simulink model "TFMMIoTSimAR"  (R2019b)
settings: Solver=VariableStepAuto  StartTime=0.0  StopTime=10  RelTol=1e-3
StartFcn:
  | startTimeStamp = num2str(posixtime(datetime('now')) * 1e6);
  | disp(strcat("Script Start: ", startTimeStamp));
  | cont = 0;
StopFcn:
  | topicMovAux = strcat(topicMov, "/Details");
  | timeStamp = num2str(posixtime(datetime('now')) * 1e6);
  | disp(strcat("Script End: ", timeStamp));
  | 
  | %Mensaje: CodigoEntrenamiento CodigoMovimiento FechaInicio FechaFin
  | msg = strcat(num2str(movCodeTrain), " ", num2str(movCode), " ", startTimeStamp, " ", timeStamp);
  | 
  | if movCodeTrain == 3
  |     msg = strcat(msg, " ", num2str(messValue));
  | end
  | 
  | publish(myMQTT, topicMovAux, msg);
model workspace (MAT data in the model file):
  gen3 = robotics.RigidBodyTree
  gen3.TreeInternal = robotics.manip.internal.RigidBodyTree
  gen3.TreeInternal.NumBodies = 8
  gen3.TreeInternal.Base = robotics.manip.internal.RigidBody
  gen3.TreeInternal.Base.Index = 0
  gen3.TreeInternal.Base.NameInternal = 'base_link'
  gen3.TreeInternal.Base.JointInternal = robotics.Joint
  gen3.TreeInternal.Base.JointInternal.Type = 'fixed'
  gen3.TreeInternal.Base.JointInternal.VelocityNumber = 0
  gen3.TreeInternal.Base.JointInternal.PositionNumber = 0
  gen3.TreeInternal.Base.JointInternal.MotionSubspace = [0; 0; 0; 0; 0; 0]
  gen3.TreeInternal.Base.JointInternal.NameInternal = 'base_link_jnt'
  gen3.TreeInternal.Base.ParentIndex = -1
  gen3.TreeInternal.Base.ChildrenIndices = 1
  gen3.TreeInternal.Base.MassInternal = 1.661
  gen3.TreeInternal.Base.CenterOfMassInternal = [-0.00077898 -4.2629e-05 0.077301]
  gen3.TreeInternal.Base.InertiaInternal = [0.0146026165007  -3.37077056916e-07  5.17806646798e-05; -3.37077056916e-07  0.0146456213934  1.24353405047e-06; 5.17806646798e-05  1.24353405047e-06  0.00199681092957]
  gen3.TreeInternal.Base.SpatialInertia = [0.0146026165007  -3.37077056916e-07  5.17806646798e-05  0  -0.128396961  -7.0806769e-05; -3.37077056916e-07  0.0146456213934  1.24353405047e-06  0.128396961  0  0.00129388578; 5.17806646798e-05  1.24353405047e-06  0.00199681092957  7.0806769e-05  -0.00129388578  0; 0  0.128396961  7.0806769e-05  1.661  0  0; -0.128396961  0  -0.00129388578  0  1.661  0; -7.0806769e-05  0.00129388578  0  0  0  1.661]
  gen3.TreeInternal.Base.VisualsInternal{1} = robotics.manip.internal.RigidBodyGeometry
  gen3.TreeInternal.Base.VisualsInternal{1}.SourceData = {'Mesh', '/mathworks/devel/bat/Brobot/build/matlab/toolbox/robotics/robotmanip/data/kortex_description/meshes/base_link.STL'}
  gen3.TreeInternal.Base.VisualsInternal{1}.Vertices = [0.0238897390664 0.0238897390664 0.0248048026115 0.0248048026115 0.0260548014194 0.0260548014194 0.0273048020899 0.0273048020899 0.028219865635 0.028219865635 0.0285465624183 0.0285548008978 ... (5268 elements, 1756x3)]
  gen3.TreeInternal.Base.VisualsInternal{1}.Faces = [1 3 3 5 5 7 7 8 9 9 12 12 ... (10362 elements, 3454x3)]
  gen3.TreeInternal.Base.VisualsInternal{1}.Color = [0.79216 0.81961 0.93333 1]
  gen3.TreeInternal.Base.VisualsInternal{1}.Tform = [1  0  0  0; 0  1  0  0; 0  0  1  0; 0  0  0  1]
  gen3.TreeInternal.Gravity = [0 0 -9.81]
  gen3.TreeInternal.Bodies{1} = robotics.manip.internal.RigidBody
  gen3.TreeInternal.Bodies{1}.Index = 1
  gen3.TreeInternal.Bodies{1}.NameInternal = 'Shoulder_Link'
  gen3.TreeInternal.Bodies{1}.JointInternal = robotics.Joint
  gen3.TreeInternal.Bodies{1}.JointInternal.Type = 'revolute'
  gen3.TreeInternal.Bodies{1}.JointInternal.VelocityNumber = 1
  gen3.TreeInternal.Bodies{1}.JointInternal.PositionNumber = 1
  gen3.TreeInternal.Bodies{1}.JointInternal.MotionSubspace = [0; 0; 1; 0; 0; 0]
  gen3.TreeInternal.Bodies{1}.JointInternal.InTree = 1
  gen3.TreeInternal.Bodies{1}.JointInternal.JointToParentTransform = [1  0  0  0; 0  -0.999999999973  7.34641020664e-06  0; 0  -7.34641020664e-06  -0.999999999973  0.15643; 0  0  0  1]
  gen3.TreeInternal.Bodies{1}.JointInternal.NameInternal = 'Actuator1'
  gen3.TreeInternal.Bodies{1}.JointInternal.PositionLimitsInternal = [-Inf Inf]
  gen3.TreeInternal.Bodies{1}.JointInternal.JointAxisInternal = [0 0 1]
  gen3.TreeInternal.Bodies{1}.ParentIndex = 0
  gen3.TreeInternal.Bodies{1}.ChildrenIndices = [0 1]
  gen3.TreeInternal.Bodies{1}.MassInternal = 2.009
  gen3.TreeInternal.Bodies{1}.CenterOfMassInternal = [-2.2888e-05 -0.010511 -0.075159]
  gen3.TreeInternal.Bodies{1}.InertiaInternal = [0.0160786470116  -1.34157671791e-06  -5.35566053673e-06; -1.34157671791e-06  0.016118091492  -0.00204244246424; -5.35566053673e-06  -0.00204244246424  0.00161225762452]
  gen3.TreeInternal.Bodies{1}.SpatialInertia = [0.0160786470116  -1.34157671791e-06  -5.35566053673e-06  0  0.150994431  -0.021116599; -1.34157671791e-06  0.016118091492  -0.00204244246424  -0.150994431  0  4.5981992e-05; -5.35566053673e-06  -0.00204244246424  0.00161225762452  0.021116599  -4.5981992e-05  0; 0  -0.150994431  0.021116599  2.009  0  0; 0.150994431  0  -4.5981992e-05  0  2.009  0; -0.021116599  4.5981992e-05  0  0  0  2.009]
  gen3.TreeInternal.Bodies{1}.VisualsInternal{1} = robotics.manip.internal.RigidBodyGeometry
  gen3.TreeInternal.Bodies{1}.VisualsInternal{1}.SourceData = {'Mesh', '/mathworks/devel/bat/Brobot/build/matlab/toolbox/robotics/robotmanip/data/kortex_description/meshes/Shoulder_Link.STL'}
  gen3.TreeInternal.Bodies{1}.VisualsInternal{1}.Vertices = [-0.00565051892772 0.000944308878388 0.000944308878388 0.00751337828115 0.00751337828115 0.0138775017112 0.0138775017112 0.0198630858213 0.0198630858213 0.0253068543971 0.0253068543971 0.03006031923 ... (14295 elements, 4765x3)]
  gen3.TreeInternal.Bodies{1}.VisualsInternal{1}.Faces = [1 3 3 5 5 7 7 9 9 11 11 13 ... (28566 elements, 9522x3)]
  gen3.TreeInternal.Bodies{1}.VisualsInternal{1}.Color = [0.86667 0.86667 0.8902 1]
  gen3.TreeInternal.Bodies{1}.VisualsInternal{1}.Tform = [1  0  0  0; 0  1  0  0; 0  0  1  0; 0  0  0  1]
  gen3.TreeInternal.Bodies{2} = robotics.manip.internal.RigidBody
  gen3.TreeInternal.Bodies{2}.Index = 2
  gen3.TreeInternal.Bodies{2}.NameInternal = 'HalfArm1_Link'
  gen3.TreeInternal.Bodies{2}.JointInternal = robotics.Joint
  gen3.TreeInternal.Bodies{2}.JointInternal.Type = 'revolute'
  gen3.TreeInternal.Bodies{2}.JointInternal.VelocityNumber = 1
  gen3.TreeInternal.Bodies{2}.JointInternal.PositionNumber = 1
  gen3.TreeInternal.Bodies{2}.JointInternal.MotionSubspace = [0; 0; 1; 0; 0; 0]
  gen3.TreeInternal.Bodies{2}.JointInternal.InTree = 1
  gen3.TreeInternal.Bodies{2}.JointInternal.JointToParentTransform = [1  0  0  0; 0  -3.67320510335e-06  -0.999999999993  0.005375; 0  0.999999999993  -3.67320510335e-06  -0.12838; 0  0  0  1]
  gen3.TreeInternal.Bodies{2}.JointInternal.NameInternal = 'Actuator2'
  gen3.TreeInternal.Bodies{2}.JointInternal.PositionLimitsInternal = [-2.2 2.2]
  gen3.TreeInternal.Bodies{2}.JointInternal.JointAxisInternal = [0 0 1]
  gen3.TreeInternal.Bodies{2}.ParentIndex = 1
  gen3.TreeInternal.Bodies{2}.ChildrenIndices = [0 0 1]
  gen3.TreeInternal.Bodies{2}.MassInternal = 1.106
  gen3.TreeInternal.Bodies{2}.CenterOfMassInternal = [-2.7821e-05 -0.097298 -0.012693]
  gen3.TreeInternal.Bodies{2}.InertiaInternal = [0.0195653824366  -5.89336198975e-06  -5.56983940018e-07; -5.89336198975e-06  0.000909251003447  -0.000848233886484; -5.56983940018e-07  -0.000848233886484  0.0195119931453]
  gen3.TreeInternal.Bodies{2}.SpatialInertia = [0.0195653824366  -5.89336198975e-06  -5.56983940018e-07  0  0.014038458  -0.107611588; -5.89336198975e-06  0.000909251003447  -0.000848233886484  -0.014038458  0  3.0770026e-05; -5.56983940018e-07  -0.000848233886484  0.0195119931453  0.107611588  -3.0770026e-05  0; 0  -0.014038458  0.107611588  1.106  0  0; 0.014038458  0  -3.0770026e-05  0  1.106  0; -0.107611588  3.0770026e-05  0  0  0  1.106]
  gen3.TreeInternal.Bodies{2}.VisualsInternal{1} = robotics.manip.internal.RigidBodyGeometry
  gen3.TreeInternal.Bodies{2}.VisualsInternal{1}.SourceData = {'Mesh', '/mathworks/devel/bat/Brobot/build/matlab/toolbox/robotics/robotmanip/data/kortex_description/meshes/HalfArm1_Link.STL'}
  gen3.TreeInternal.Bodies{2}.VisualsInternal{1}.Vertices = [-0.00426170928404 -0.0107498951256 -0.0107498951256 -0.0169448517263 -0.0169448517263 -0.0226775947958 -0.0226775947958 -0.0277917552739 -0.0277917552739 -0.0321478284895 -0.0321478284895 -0.0356269925833 ... (15435 elements, 5145x3)]
  gen3.TreeInternal.Bodies{2}.VisualsInternal{1}.Faces = [1 3 3 5 5 7 7 9 9 11 11 13 ... (30846 elements, 10282x3)]
  gen3.TreeInternal.Bodies{2}.VisualsInternal{1}.Color = [0.89804 0.91765 0.92941 1]
  gen3.TreeInternal.Bodies{2}.VisualsInternal{1}.Tform = [1  0  0  0; 0  1  0  0; 0  0  1  0; 0  0  0  1]
  gen3.TreeInternal.Bodies{3} = robotics.manip.internal.RigidBody
  gen3.TreeInternal.Bodies{3}.Index = 3
  gen3.TreeInternal.Bodies{3}.NameInternal = 'HalfArm2_Link'
  gen3.TreeInternal.Bodies{3}.JointInternal = robotics.Joint
  gen3.TreeInternal.Bodies{3}.JointInternal.Type = 'revolute'
  gen3.TreeInternal.Bodies{3}.JointInternal.VelocityNumber = 1
  gen3.TreeInternal.Bodies{3}.JointInternal.PositionNumber = 1
  gen3.TreeInternal.Bodies{3}.JointInternal.MotionSubspace = [0; 0; 1; 0; 0; 0]
  gen3.TreeInternal.Bodies{3}.JointInternal.InTree = 1
  gen3.TreeInternal.Bodies{3}.JointInternal.JointToParentTransform = [1  0  0  0; 0  -3.67320510335e-06  0.999999999993  -0.21038; 0  -0.999999999993  -3.67320510335e-06  -0.006375; 0  0  0  1]
  gen3.TreeInternal.Bodies{3}.JointInternal.NameInternal = 'Actuator3'
  gen3.TreeInternal.Bodies{3}.JointInternal.PositionLimitsInternal = [-Inf Inf]
  gen3.TreeInternal.Bodies{3}.JointInternal.JointAxisInternal = [0 0 1]
  gen3.TreeInternal.Bodies{3}.ParentIndex = 2
  gen3.TreeInternal.Bodies{3}.ChildrenIndices = [0 0 0 1]
  gen3.TreeInternal.Bodies{3}.MassInternal = 1.106
  gen3.TreeInternal.Bodies{3}.CenterOfMassInternal = [2.9808e-05 -0.0062391 -0.11552]
  gen3.TreeInternal.Bodies{3}.InertiaInternal = [0.0236731792263  4.40038452637e-07  4.8822269696e-07; 4.40038452637e-07  0.0237628276451  -0.00130128936019; 4.8822269696e-07  -0.00130128936019  0.000761643546604]
  gen3.TreeInternal.Bodies{3}.SpatialInertia = [0.0236731792263  4.40038452637e-07  4.8822269696e-07  0  0.12776512  -0.0069004446; 4.40038452637e-07  0.0237628276451  -0.00130128936019  -0.12776512  0  -3.2967648e-05; 4.8822269696e-07  -0.00130128936019  0.000761643546604  0.0069004446  3.2967648e-05  0; 0  -0.12776512  0.0069004446  1.106  0  0; 0.12776512  0  3.2967648e-05  0  1.106  0; -0.0069004446  -3.2967648e-05  0  0  0  1.106]
  gen3.TreeInternal.Bodies{3}.VisualsInternal{1} = robotics.manip.internal.RigidBodyGeometry
  gen3.TreeInternal.Bodies{3}.VisualsInternal{1}.SourceData = {'Mesh', '/mathworks/devel/bat/Brobot/build/matlab/toolbox/robotics/robotmanip/data/kortex_description/meshes/HalfArm2_Link.STL'}
  gen3.TreeInternal.Bodies{3}.VisualsInternal{1}.Vertices = [0.0415250770748 0.0427930280566 0.0435288511217 0.0452561341226 0.0460000932217 0.0459154732525 -0.0121358856559 -0.00814644899219 -0.00789992138743 -0.0130066424608 -0.00873851031065 -0.00857216585428 ... (14685 elements, 4895x3)]
  gen3.TreeInternal.Bodies{3}.VisualsInternal{1}.Faces = [1 4 7 10 13 12 17 20 23 26 29 32 ... (29346 elements, 9782x3)]
  gen3.TreeInternal.Bodies{3}.VisualsInternal{1}.Color = [0.89804 0.91765 0.92941 1]
  gen3.TreeInternal.Bodies{3}.VisualsInternal{1}.Tform = [1  0  0  0; 0  1  0  0; 0  0  1  0; 0  0  0  1]
  gen3.TreeInternal.Bodies{4} = robotics.manip.internal.RigidBody
  gen3.TreeInternal.Bodies{4}.Index = 4
  gen3.TreeInternal.Bodies{4}.NameInternal = 'ForeArm_Link'
  gen3.TreeInternal.Bodies{4}.JointInternal = robotics.Joint
  gen3.TreeInternal.Bodies{4}.JointInternal.Type = 'revolute'
  gen3.TreeInternal.Bodies{4}.JointInternal.VelocityNumber = 1
  gen3.TreeInternal.Bodies{4}.JointInternal.PositionNumber = 1
  gen3.TreeInternal.Bodies{4}.JointInternal.MotionSubspace = [0; 0; 1; 0; 0; 0]
  gen3.TreeInternal.Bodies{4}.JointInternal.InTree = 1
  gen3.TreeInternal.Bodies{4}.JointInternal.JointToParentTransform = [1  0  0  0; 0  -3.67320510335e-06  -0.999999999993  0.006375; 0  0.999999999993  -3.67320510335e-06  -0.21038; 0  0  0  1]
  gen3.TreeInternal.Bodies{4}.JointInternal.NameInternal = 'Actuator4'
  gen3.TreeInternal.Bodies{4}.JointInternal.PositionLimitsInternal = [-2.5656 2.5656]
  gen3.TreeInternal.Bodies{4}.JointInternal.JointAxisInternal = [0 0 1]
  gen3.TreeInternal.Bodies{4}.ParentIndex = 3
  gen3.TreeInternal.Bodies{4}.ChildrenIndices = [0 0 0 0 1]
  gen3.TreeInternal.Bodies{4}.MassInternal = 0.895
  gen3.TreeInternal.Bodies{4}.CenterOfMassInternal = [-1.1024e-05 -0.075357 -0.014085]
  gen3.TreeInternal.Bodies{4}.InertiaInternal = [0.0119938728832  -4.704833336e-08  -1.613933708e-07; -4.704833336e-08  0.000628436675143  -0.000559965993775; -1.613933708e-07  -0.000559965993775  0.0119437164256]
  gen3.TreeInternal.Bodies{4}.SpatialInertia = [0.0119938728832  -4.704833336e-08  -1.613933708e-07  0  0.012606075  -0.067444515; -4.704833336e-08  0.000628436675143  -0.000559965993775  -0.012606075  0  9.86648e-06; -1.613933708e-07  -0.000559965993775  0.0119437164256  0.067444515  -9.86648e-06  0; 0  -0.012606075  0.067444515  0.895  0  0; 0.012606075  0  -9.86648e-06  0  0.895  0; -0.067444515  9.86648e-06  0  0  0  0.895]
  gen3.TreeInternal.Bodies{4}.VisualsInternal{1} = robotics.manip.internal.RigidBodyGeometry
  gen3.TreeInternal.Bodies{4}.VisualsInternal{1}.SourceData = {'Mesh', '/mathworks/devel/bat/Brobot/build/matlab/toolbox/robotics/robotmanip/data/kortex_description/meshes/ForeArm_Link.STL'}
  gen3.TreeInternal.Bodies{4}.VisualsInternal{1}.Vertices = [0.00536897266284 8.53809210832e-18 7.61652026171e-18 0.0168247949332 0.0172408241779 0.00878553558141 0.0446321181953 0.0425008013844 0.0423283949494 0.0287076402456 0.0292822066694 0.0347713828087 ... (13698 elements, 4566x3)]
  gen3.TreeInternal.Bodies{4}.VisualsInternal{1}.Faces = [1 4 7 10 13 16 19 22 25 28 31 3 ... (27372 elements, 9124x3)]
  gen3.TreeInternal.Bodies{4}.VisualsInternal{1}.Color = [0.79216 0.81961 0.93333 1]
  gen3.TreeInternal.Bodies{4}.VisualsInternal{1}.Tform = [1  0  0  0; 0  1  0  0; 0  0  1  0; 0  0  0  1]
  gen3.TreeInternal.Bodies{5} = robotics.manip.internal.RigidBody
  gen3.TreeInternal.Bodies{5}.Index = 5
  gen3.TreeInternal.Bodies{5}.NameInternal = 'Wrist1_Link'
  gen3.TreeInternal.Bodies{5}.JointInternal = robotics.Joint
  gen3.TreeInternal.Bodies{5}.JointInternal.Type = 'revolute'
  gen3.TreeInternal.Bodies{5}.JointInternal.VelocityNumber = 1
  gen3.TreeInternal.Bodies{5}.JointInternal.PositionNumber = 1
  gen3.TreeInternal.Bodies{5}.JointInternal.MotionSubspace = [0; 0; 1; 0; 0; 0]
  gen3.TreeInternal.Bodies{5}.JointInternal.InTree = 1
  gen3.TreeInternal.Bodies{5}.JointInternal.JointToParentTransform = [1  0  0  0; 0  -3.67320510335e-06  0.999999999993  -0.20843; 0  -0.999999999993  -3.67320510335e-06  -0.006375; 0  0  0  1]
  gen3.TreeInternal.Bodies{5}.JointInternal.NameInternal = 'Actuator5'
  gen3.TreeInternal.Bodies{5}.JointInternal.PositionLimitsInternal = [-Inf Inf]
  gen3.TreeInternal.Bodies{5}.JointInternal.JointAxisInternal = [0 0 1]
  gen3.TreeInternal.Bodies{5}.ParentIndex = 4
  gen3.TreeInternal.Bodies{5}.ChildrenIndices = [0 0 0 0 0 1]
  gen3.TreeInternal.Bodies{5}.MassInternal = 0.654
  gen3.TreeInternal.Bodies{5}.CenterOfMassInternal = [-3.2964e-07 -0.009617 -0.062968]
  gen3.TreeInternal.Bodies{5}.InertiaInternal = [0.0039846760363  -2.53176671352e-09  -1.40017085741e-08; -2.53176671352e-09  0.00392128974177  -0.000625398369424; -1.40017085741e-08  -0.000625398369424  0.000367446294677]
  gen3.TreeInternal.Bodies{5}.SpatialInertia = [0.0039846760363  -2.53176671352e-09  -1.40017085741e-08  0  0.041181072  -0.006289518; -2.53176671352e-09  0.00392128974177  -0.000625398369424  -0.041181072  0  2.1558456e-07; -1.40017085741e-08  -0.000625398369424  0.000367446294677  0.006289518  -2.1558456e-07  0; 0  -0.041181072  0.006289518  0.654  0  0; 0.041181072  0  -2.1558456e-07  0  0.654  0; -0.006289518  2.1558456e-07  0  0  0  0.654]
  gen3.TreeInternal.Bodies{5}.VisualsInternal{1} = robotics.manip.internal.RigidBodyGeometry
  gen3.TreeInternal.Bodies{5}.VisualsInternal{1}.SourceData = {'Mesh', '/mathworks/devel/bat/Brobot/build/matlab/toolbox/robotics/robotmanip/data/kortex_description/meshes/Wrist1_Link.STL'}
  gen3.TreeInternal.Bodies{5}.VisualsInternal{1}.Vertices = [-0.03472366184 -0.0341793373227 -0.0341129377484 -0.00542340660468 -0.00378200318664 1.25496401465e-17 -0.00703497463837 -0.0103659555316 -0.0106233013794 -0.0106383524835 -0.0155325094238 -0.0111691672355 ... (16404 elements, 5468x3)]
  gen3.TreeInternal.Bodies{5}.VisualsInternal{1}.Faces = [1 4 7 4 4 11 10 11 11 15 16 17 ... (32784 elements, 10928x3)]
  gen3.TreeInternal.Bodies{5}.VisualsInternal{1}.Color = [0.79216 0.81961 0.93333 1]
  gen3.TreeInternal.Bodies{5}.VisualsInternal{1}.Tform = [1  0  0  0; 0  1  0  0; 0  0  1  0; 0  0  0  1]
  gen3.TreeInternal.Bodies{6} = robotics.manip.internal.RigidBody
  gen3.TreeInternal.Bodies{6}.Index = 6
  gen3.TreeInternal.Bodies{6}.NameInternal = 'Wrist2_Link'
  gen3.TreeInternal.Bodies{6}.JointInternal = robotics.Joint
  gen3.TreeInternal.Bodies{6}.JointInternal.Type = 'revolute'
  gen3.TreeInternal.Bodies{6}.JointInternal.VelocityNumber = 1
  gen3.TreeInternal.Bodies{6}.JointInternal.PositionNumber = 1
  gen3.TreeInternal.Bodies{6}.JointInternal.MotionSubspace = [0; 0; 1; 0; 0; 0]
  gen3.TreeInternal.Bodies{6}.JointInternal.InTree = 1
  gen3.TreeInternal.Bodies{6}.JointInternal.JointToParentTransform = [1  0  0  0; 0  -3.67320510335e-06  -0.999999999993  0.00017505; 0  0.999999999993  -3.67320510335e-06  -0.10593; 0  0  0  1]
  gen3.TreeInternal.Bodies{6}.JointInternal.NameInternal = 'Actuator6'
  gen3.TreeInternal.Bodies{6}.JointInternal.PositionLimitsInternal = [-2.05 2.05]
  gen3.TreeInternal.Bodies{6}.JointInternal.JointAxisInternal = [0 0 1]
  gen3.TreeInternal.Bodies{6}.ParentIndex = 5
  gen3.TreeInternal.Bodies{6}.ChildrenIndices = [0 0 0 0 0 0 1]
  gen3.TreeInternal.Bodies{6}.MassInternal = 0.654
  gen3.TreeInternal.Bodies{6}.CenterOfMassInternal = [-3.4377e-07 -0.044043 -0.0097804]
  gen3.TreeInternal.Bodies{6}.InertiaInternal = [0.00267337911585  -9.40603301994e-09  -2.93270410263e-09; -9.40603301994e-09  0.000372809170678  -4.66558348088e-05; -2.93270410263e-09  -4.66558348088e-05  0.00260461994532]
  gen3.TreeInternal.Bodies{6}.SpatialInertia = [0.00267337911585  -9.40603301994e-09  -2.93270410263e-09  0  0.0063963816  -0.028804122; -9.40603301994e-09  0.000372809170678  -4.66558348088e-05  -0.0063963816  0  2.2482558e-07; -2.93270410263e-09  -4.66558348088e-05  0.00260461994532  0.028804122  -2.2482558e-07  0; 0  -0.0063963816  0.028804122  0.654  0  0; 0.0063963816  0  -2.2482558e-07  0  0.654  0; -0.028804122  2.2482558e-07  0  0  0  0.654]
  gen3.TreeInternal.Bodies{6}.VisualsInternal{1} = robotics.manip.internal.RigidBodyGeometry
  gen3.TreeInternal.Bodies{6}.VisualsInternal{1}.SourceData = {'Mesh', '/mathworks/devel/bat/Brobot/build/matlab/toolbox/robotics/robotmanip/data/kortex_description/meshes/Wrist2_Link.STL'}
  gen3.TreeInternal.Bodies{6}.VisualsInternal{1}.Vertices = [-0.0139686269686 -0.0139704411849 -0.0135804964229 -0.00560790300369 -5.85475678355e-14 -0.00356922904029 -5.85477304658e-14 -0.0103755732998 -0.0109685873613 -0.0109075605869 -0.0118341417983 -0.0135629465804 ... (15519 elements, 5173x3)]
  gen3.TreeInternal.Bodies{6}.VisualsInternal{1}.Faces = [1 4 6 8 10 10 13 16 18 18 21 18 ... (31014 elements, 10338x3)]
  gen3.TreeInternal.Bodies{6}.VisualsInternal{1}.Color = [0.79216 0.81961 0.93333 1]
  gen3.TreeInternal.Bodies{6}.VisualsInternal{1}.Tform = [1  0  0  0; 0  1  0  0; 0  0  1  0; 0  0  0  1]
  gen3.TreeInternal.Bodies{7} = robotics.manip.internal.RigidBody
  gen3.TreeInternal.Bodies{7}.Index = 7
  gen3.TreeInternal.Bodies{7}.NameInternal = 'Bracelet_Link'
  gen3.TreeInternal.Bodies{7}.JointInternal = robotics.Joint
  gen3.TreeInternal.Bodies{7}.JointInternal.Type = 'revolute'
  gen3.TreeInternal.Bodies{7}.JointInternal.VelocityNumber = 1
  gen3.TreeInternal.Bodies{7}.JointInternal.PositionNumber = 1
  gen3.TreeInternal.Bodies{7}.JointInternal.MotionSubspace = [0; 0; 1; 0; 0; 0]
  gen3.TreeInternal.Bodies{7}.JointInternal.InTree = 1
  gen3.TreeInternal.Bodies{7}.JointInternal.JointToParentTransform = [1  0  0  0; 0  -3.67320510335e-06  0.999999999993  -0.10593; 0  -0.999999999993  -3.67320510335e-06  -0.00017505; 0  0  0  1]
  gen3.TreeInternal.Bodies{7}.JointInternal.NameInternal = 'Actuator7'
  gen3.TreeInternal.Bodies{7}.JointInternal.PositionLimitsInternal = [-Inf Inf]
  gen3.TreeInternal.Bodies{7}.JointInternal.JointAxisInternal = [0 0 1]
  gen3.TreeInternal.Bodies{7}.ParentIndex = 6
  gen3.TreeInternal.Bodies{7}.ChildrenIndices = [0 0 0 0 0 0 0 1]
  gen3.TreeInternal.Bodies{7}.MassInternal = 0.31408
  gen3.TreeInternal.Bodies{7}.CenterOfMassInternal = [-2.788e-05 -0.0052162 -0.022692]
  gen3.TreeInternal.Bodies{7}.InertiaInternal = [0.000396673951271  -5.36585918196e-07  -4.61083641677e-07; -5.36585918196e-07  0.000318698473578  -8.27903965464e-05; -4.61083641677e-07  -8.27903965464e-05  0.000268355965958]
  gen3.TreeInternal.Bodies{7}.SpatialInertia = [0.000396673951271  -5.36585918196e-07  -4.61083641677e-07  0  0.00712710336  -0.001638304096; -5.36585918196e-07  0.000318698473578  -8.27903965464e-05  -0.00712710336  0  8.7565504e-06; -4.61083641677e-07  -8.27903965464e-05  0.000268355965958  0.001638304096  -8.7565504e-06  0; 0  -0.00712710336  0.001638304096  0.31408  0  0; 0.00712710336  0  -8.7565504e-06  0  0.31408  0; -0.001638304096  8.7565504e-06  0  0  0  0.31408]
  gen3.TreeInternal.Bodies{7}.VisualsInternal{1} = robotics.manip.internal.RigidBodyGeometry
  gen3.TreeInternal.Bodies{7}.VisualsInternal{1}.SourceData = {'Mesh', '/mathworks/devel/bat/Brobot/build/matlab/toolbox/robotics/robotmanip/data/kortex_description/meshes/Bracelet_Link.STL'}
  gen3.TreeInternal.Bodies{7}.VisualsInternal{1}.Vertices = [0.012051442638 0.011827503331 0.00789115857333 0.0124131245539 0.0117499995977 0.0117499995977 0.00790539011359 0.0118271494284 0.012051442638 0.0124130398035 0.0128750000149 0.0139628034085 ... (34896 elements, 11632x3)]
  gen3.TreeInternal.Bodies{7}.VisualsInternal{1}.Faces = [1 1 5 7 7 9 7 7 12 12 15 14 ... (69888 elements, 23296x3)]
  gen3.TreeInternal.Bodies{7}.VisualsInternal{1}.Color = [0.79216 0.81961 0.93333 1]
  gen3.TreeInternal.Bodies{7}.VisualsInternal{1}.Tform = [1  0  0  0; 0  1  0  0; 0  0  1  0; 0  0  0  1]
  gen3.TreeInternal.Bodies{8} = robotics.manip.internal.RigidBody
  gen3.TreeInternal.Bodies{8}.Index = 8
  gen3.TreeInternal.Bodies{8}.NameInternal = 'EndEffector_Link'
  gen3.TreeInternal.Bodies{8}.JointInternal = robotics.Joint
  gen3.TreeInternal.Bodies{8}.JointInternal.Type = 'fixed'
  gen3.TreeInternal.Bodies{8}.JointInternal.VelocityNumber = 0
  gen3.TreeInternal.Bodies{8}.JointInternal.PositionNumber = 0
  gen3.TreeInternal.Bodies{8}.JointInternal.MotionSubspace = [0; 0; 0; 0; 0; 0]
  gen3.TreeInternal.Bodies{8}.JointInternal.InTree = 1
  gen3.TreeInternal.Bodies{8}.JointInternal.JointToParentTransform = [1  0  0  0; 0  -0.999999999973  7.34641020664e-06  0; 0  -7.34641020664e-06  -0.999999999973  -0.059525; 0  0  0  1]
  gen3.TreeInternal.Bodies{8}.JointInternal.NameInternal = 'Endeffector'
  gen3.TreeInternal.Bodies{8}.ParentIndex = 7
  gen3.TreeInternal.Bodies{8}.ChildrenIndices = [0 0 0 0 0 0 0]
  gen3.TreeInternal.Bodies{8}.MassInternal = 0
  gen3.TreeInternal.Bodies{8}.CenterOfMassInternal = [-0.00017492 0.014824 -0.62969]
  gen3.TreeInternal.Bodies{8}.InertiaInternal = [0  0  0; 0  0  0; 0  0  0]
  gen3.TreeInternal.Bodies{8}.SpatialInertia = [0  0  0  0  0  0; 0  0  0  0  0  0; 0  0  0  0  0  0; 0  0  0  0  0  0; 0  0  0  0  0  0; 0  0  0  0  0  0]
  gen3.TreeInternal.NumNonFixedBodies = 7
  gen3.TreeInternal.PositionNumber = 7
  gen3.TreeInternal.VelocityNumber = 7
  gen3.TreeInternal.PositionDoFMap = [1  1; 2  2; 3  3; 4  4; 5  5; 6  6; 7  7; 0  -1]
  gen3.TreeInternal.VelocityDoFMap = [1  1; 2  2; 3  3; 4  4; 5  5; 6  6; 7  7; 0  -1]
  gen3.TreeInternal.MaxNumBodies = 8
  gen3.TreeInternal.MaxNameLength = 200
  gen3.TreeInternal.MaxJointPositionNumber = 7
  gen3.TreeInternal.VisualizationInfo = robotics.manip.internal.VisualizationInfo
  gen3.TreeInternal.VisualizationInfo.ShowTag = 'DO_NOT_EDIT_i93au'
  gen3.TreeInternal.DataFormatInternal = 'row___'
values from neighbouring files (symbols this model uses):
  accPoints = zeros(7, numPoints)    [TFMMIoTMain.m]
  fext = externalForce(robot,'tool0',wrench,q)    [TFMMIoTMain.m]
  messValue = 0.5    [TFMMIoTMain.m]
  numPoints = 7    [TFMMIoTMain.m]
  topicMov = 'dobot/movimiento'    [TFMMIoTMain.m]
  velPoints = ones(7, numPoints) .* messValue    [TFMMIoTMain.m]
  wayPoints = wayPointsSec01    [TFMMIoTMain.m]
libraries: vrlib x3, robotcorelib x2, robotmaniplib x2
settings Model: PauseTimes=3  EnablePacing=on  Creator=The MathWorks, Inc.  LastModifiedBy=Richard
settings DebuggingCC: SymbolicDimsDataTypeCodeGenerationDiagnostic=none

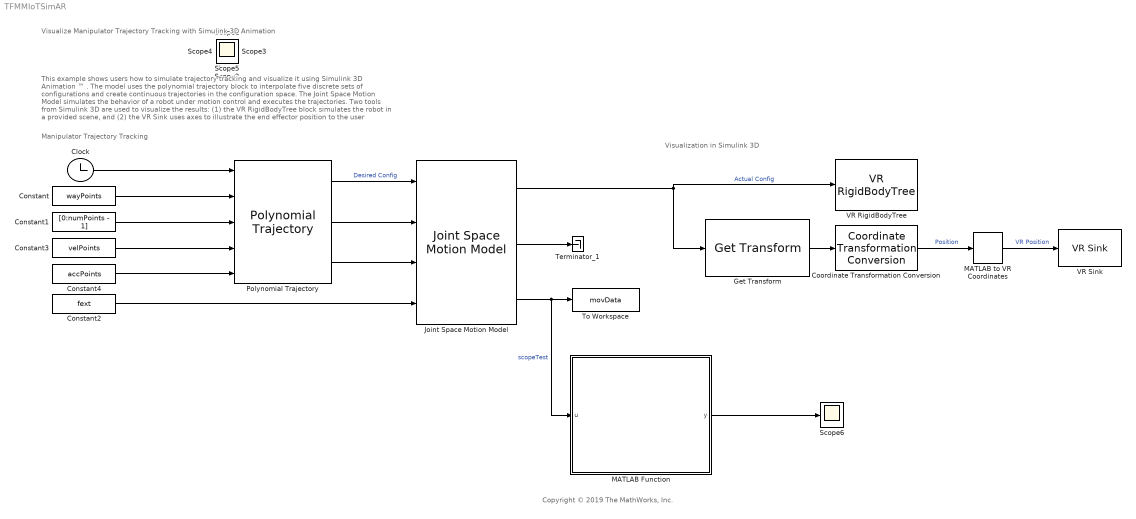
== system TFMMIoTSimAR ==
  note: This example shows users how to simulate trajectory tracking and visualize it using Simulink 3D Animation ™ . The model uses the polynomial trajectory block to interpolate five discrete sets of configurations and create continuous trajectories in the configuration space. The Joint Space Motion Model simulates the behavior of a robot under motion control and executes the trajectories. Two tools from Simulink 3D are used to visualize the results: (1) the VR RigidBodyTree block simulates the robot in a provided scene, and (2) the VR Sink uses axes to illustrate the end effector position to the user
  note: Visualize Manipulator Trajectory Tracking with Simulink 3D Animation
  note: Visualization in Simulink 3D
  note: Manipulator Trajectory Tracking
  note: Copyright © 2019 The MathWorks, Inc.
  Clock : Clock
  Constant : Constant  Value=wayPoints  VectorParams1D=off
  Constant1 : Constant  Value=[0:numPoints - 1]  VectorParams1D=off
  Constant2 : Constant  Value=fext  VectorParams1D=off
  Constant3 : Constant  Value=velPoints  VectorParams1D=off
  Constant4 : Constant  Value=accPoints  VectorParams1D=off
  Coordinate Transformation Conversion : robotcorelib/Coordinate Transformation Conversion  InputRepresentation=Homogeneous Transformation  InputEulerSequence=ZYX  ShowTrVecInputPort=on  OutputRepresentation=Translation Vector  OutputEulerSequence=ZYX  ShowTrVecOutputPort=on  SimulateUsing=Interpreted execution
      settings: SourceProductBaseCode=RO
  Get Transform : robotmaniplib/Get Transform  RigidBodyTree=gen3  SourceBody=EndEffector_Link  TargetBody=base_link  SimulateUsing=Interpreted execution
      settings: SourceProductName=Robotics System Toolbox
  Joint Space Motion Model : robotmaniplib/Joint Space Motion Model  RigidBodyTree=gen3  MotionType=Computed Torque Control  ProportionalGain=100  DerivativeGain=10  ErrorDynamicsSpecification=Damping Ratio / Natural Frequency  DampingRatio=1  NaturalFrequency=10  SettlingTime=0.59  Overshoot=0  ShowExternalForcePort=on  InitConfig=0  InitJointVel=0  SimulateUsing=Interpreted execution
      settings: SourceProductName=Robotics System Toolbox  SourceProductBaseCode=RO
  MATLAB Function : MATLAB Function  TreatAsAtomicUnit=on
  MATLAB to VR Coordinates : vrlib/Utilities/MATLAB to VR Coordinates
      settings: SourceProductName=Simulink  SourceProductBaseCode=SL
  Polynomial Trajectory : robotcorelib/Polynomial Trajectory  WaypointSource=External  Waypoints=.75*pi*wayPoints - .375*pi  TimePoints=[0:numPoints - 1]  TimeInterval=[ 1, 4 ]  Method=Quintic Polynomial  ParameterSource=External  VelocityBoundaryCondition=zeros(7, numPoints)  AccelerationBoundaryCondition=zeros( 7, numPoints)  SimulateUsing=Interpreted execution
      settings: SourceProductName=Robotics System Toolbox  SourceProductBaseCode=RO
  Scope{,1..6} (7 alike) : Scope
  Terminator_1 : Terminator
  To Workspace : ToWorkspace  VariableName=movData  SaveFormat=Timeseries  SampleTime=-1
      settings: Save2DSignal=2-D array (concatenate along first dimension)
  VR RigidBodyTree : vrlib/VR RigidBodyTree  VrmlFile=robot_manipulator_scene.wrl  GroupNode=Robot_Parent  RBT=gen3  useRBT=on  Ts=-1  ForceViewerOpen=on
      settings: SourceProductName=Simulink  SourceProductBaseCode=SL
  VR Sink : vrlib/VR Sink  InstantiateOnLoad=on  SampleTime=-1  ViewEnable=on  RemoteChange=off  RemoteView=off  FieldsWritten=SetPoint.translation.3.1.1.double  WorldFileName=robot_manipulator_scene.wrl  WorldDescription=Simple Robot Scene  AutoView=on  VideoDimensions=[]  AllowVariableSize=off  FigureProperties="{'Position', 'Name', 'Viewpoint', 'CameraBound', 'CameraDirection', 'CameraPosition', 'CameraUpVector', 'ZoomFactor', 'Antialiasing', 'Headlight', 'Lighting', 'NavPanel', 'Sound', 'StatusBar', 'Stereo3D', 'Stereo3DCameraOffset', 'Stereo3DHIT', 'ToolBar', 'Textures', 'Transparency', 'Triad', 'Wireframe', 'NavZones', 'NavMode', 'NavSpeed', 'CaptureFileFormat', 'CaptureFileName', 'Record2DCompressMethod', 'Record2DCompressQuality', 'Record2D', 'Record2DFileName', 'Record2DFPS'; [5.0000000000000000e+00   9.2000000000000000e+01   5.7600000000000000e+02   3.5000000000000000e+02], 'Simple Robot Scene', 'Close View', 'on', [0.0000000000000000e+00   0.0000000000000000e+00  -1.0000000000000000e+00], [0.0000000000000000e+00   0.0000000000000000e+00   0.0000000000000000e+00], [0.0000000000000000e+00   1.0000000000000000e+00   0.0000000000000000e+00], [1.0000000000000000e+00], 'on', 'off', 'on', 'halfbar', 'on', 'on', 'off', [1.0000000149011612e-01], [0.0000000000000000e+00], 'on', 'on', 'on', 'none', 'off', 'off', 'examine', 'normal', 'tif', '%f_anim_%n.tif', 'auto', [7.5000000000000000e+01], 'off', '%f_anim_%n.avi', 'auto'}"
      settings: SourceProductName=Simulink
  wires:
  Joint Space Motion Model/1 -> Get Transform/1, VR RigidBodyTree/1  "Actual Config"
  Joint Space Motion Model/2 -> Terminator_1/1
  Joint Space Motion Model/3 -> MATLAB Function/1(u), To Workspace/1  "scopeTest"
  Get Transform/1 -> Coordinate Transformation Conversion/1
  Coordinate Transformation Conversion/1 -> MATLAB to VR Coordinates/1  "Position"
  MATLAB to VR Coordinates/1 -> VR Sink/1  "VR Position"
  Clock/1 -> Polynomial Trajectory/1
  Constant/1 -> Polynomial Trajectory/2
  Constant1/1 -> Polynomial Trajectory/3
  Polynomial Trajectory/1 -> Joint Space Motion Model/1  "Desired Config"
  Polynomial Trajectory/2 -> Joint Space Motion Model/2
  Polynomial Trajectory/3 -> Joint Space Motion Model/3
  Constant2/1 -> Joint Space Motion Model/4
  Constant3/1 -> Polynomial Trajectory/4
  Constant4/1 -> Polynomial Trajectory/5
  MATLAB Function/1(y) -> Scope6/1

== matlab function TFMMIoTSimAR/MATLAB Function ==
  data: u input; y output
function y = TFMMIoTSigSave(u) 
    coder.extrinsic('TFMMIoTSigSave')
    %disp(u)
    TFMMIoTSigSave(u);
y = u;
